simulink model "P1_LC"  (R2023b)
settings: Solver=VariableStepAuto  StartTime=0.0  StopTime=10.0  RelTol=1e-3
undefined symbols (not defined in the file): DiscIntNeverNeededParam
settings Model: Creator=Usuario_UMA  LastModifiedBy=pcele

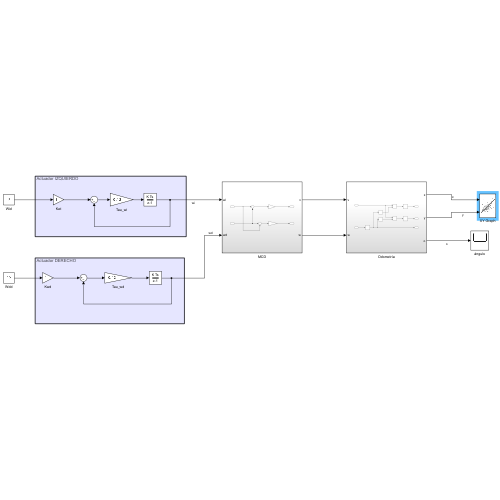
[thumbnail: Simulink's stored preview of the top-level diagram]
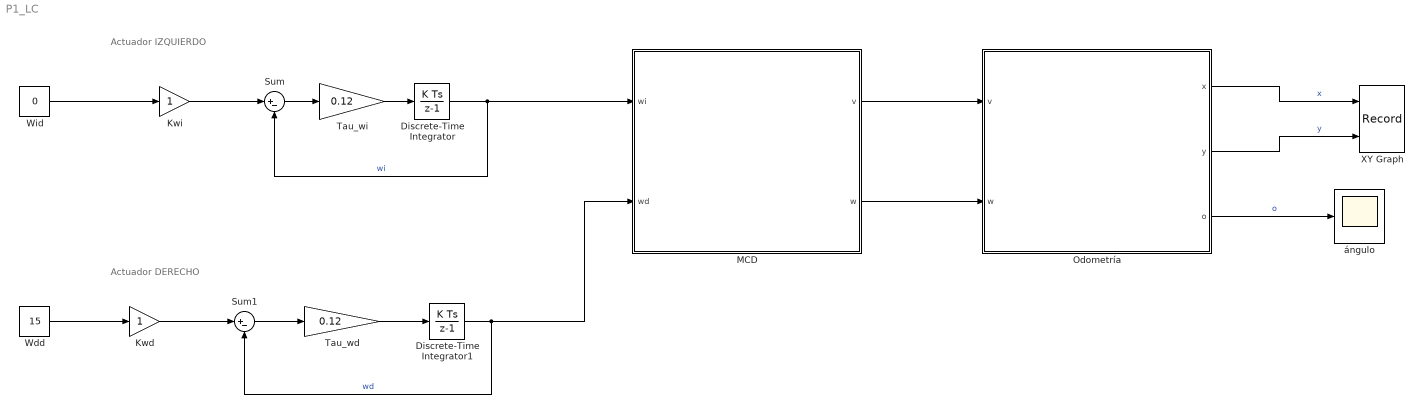
== system P1_LC ==
  note: Actuador IZQUIERDO
  note: Actuador DERECHO
  Discrete-Time Integrator : DiscreteIntegrator  SampleTime=0.25  ICPrevOutput=DiscIntNeverNeededParam  ICPrevScaledInput=DiscIntNeverNeededParam
  Discrete-Time Integrator1 : DiscreteIntegrator  SampleTime=0.25  ICPrevOutput=DiscIntNeverNeededParam  ICPrevScaledInput=DiscIntNeverNeededParam
  Kwd : Gain
  Kwi : Gain
  MCD : Subsystem
  Odometría : Subsystem
  Sum : Sum  Inputs=|+-
  Sum1 : Sum  Inputs=|+-
  Tau_wd : Gain  Gain=0.12
  Tau_wi : Gain  Gain=0.12
  Wdd : Constant  Value=15
  Wid : Constant  Value=0
  XY Graph : Record  FileSettingsInternal="{\"entries\":[{\"content\":{\"excelSettings\":{\"content\":{},\"type\":\"Streamout.ExcelSettings\"}},\"type\":\"Streamout.FileSettingStorage\",\"uuid\":\"\"}],\"packageUris\":[\"http:\\/\\/schema.mathworks.com\\/mf0\\/streamout_blocks\\/R2020a\"],\"version\":\"1.0\"}"  Layout=[1 1]  SignalsInternal="{\"entries\":[{\"content\":{\"signals\":[{\"content\":{\"blockPath\":[],\"dimensions\":[1],\"domain\":\"\",\"lineColor\":\"#a2142f\",\"plots\":[ 1 ],\"port\":1,\"sid\":[\"\"],\"signalID\":1,\"signalName\":\"x\"},\"type\":\"RecordBlkView.Signal\",\"uuid\":\"\"},{\"content\":{\"blockPath\":[],\"dimensions\":[1],\"domain\":\"\",\"lineColor\":\"#139fff\",\"plots\":[ 1 ],\"port\":2,\"sid\":[\"\"],\"signalID\":2,\"signalName\":\"y\"},\"type\":\"RecordBlkView.Signal\",\"uuid\":\"\"}]},\"type\":\"RecordBlkView.InputSignals\",\"uuid\":\"\"}],\"packageUris\":[\"http:\\/\\/schema.mathworks.com\\/mf0\\/streamout_blocks\\/R2020a\"],\"version\":\"1.0\"}"  VisualizationBindings="{\"xyplotplugin\":{\"info\":[{\"series\":[{\"bindingParametersList\":[{\"parameter\":\"X-Axis\",\"signalID\":1,\"signalName\":\"x\"},{\"parameter\":\"Y-Axis\",\"signalID\":2,\"signalName\":\"y\"}],\"seriesID\":0}],\"subplotID\":1}]}}"  CompatibilityTag=XY
  ángulo : Scope
  wires:
  Wid/1 -> Kwi/1
  Kwi/1 -> Sum/1
  Wdd/1 -> Kwd/1
  Kwd/1 -> Sum1/1
  Discrete-Time Integrator1/1 -> MCD/2(wd), Sum1/2  "wd"
  Sum1/1 -> Tau_wd/1
  Sum/1 -> Tau_wi/1
  Tau_wi/1 -> Discrete-Time Integrator/1
  Tau_wd/1 -> Discrete-Time Integrator1/1
  Discrete-Time Integrator/1 -> MCD/1(wi), Sum/2  "wi"
  MCD/1(v) -> Odometría/1(v)
  MCD/2(w) -> Odometría/2(w)
  Odometría/3(o) -> ángulo/1  "o"
  Odometría/1(x) -> XY Graph/1  "x"
  Odometría/2(y) -> XY Graph/2  "y"

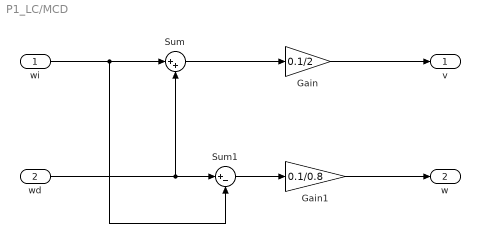
== system P1_LC/MCD ==
  wi : Inport
  wd : Inport  Port=2
  Gain : Gain  Gain=0.1/2
  Gain1 : Gain  Gain=0.1/0.8
  Sum : Sum  Inputs=|++
  Sum1 : Sum  Inputs=|+-
  v : Outport
  w : Outport  Port=2
  wires:
  Sum1/1 -> Gain1/1
  wd/1 -> Sum/2, Sum1/1
  wi/1 -> Sum1/2, Sum/1
  Sum/1 -> Gain/1
  Gain/1 -> v/1
  Gain1/1 -> w/1

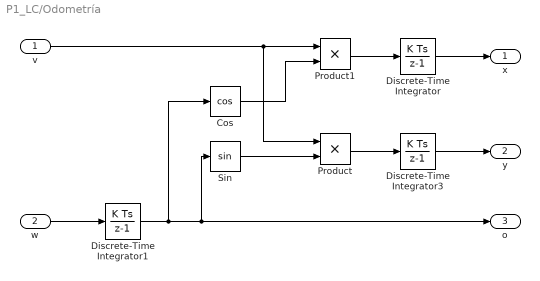
== system P1_LC/Odometría ==
  v : Inport
  w : Inport  Port=2
  Cos : Trigonometry  Operator=cos
  Discrete-Time Integrator : DiscreteIntegrator  SampleTime=0.25  ICPrevOutput=DiscIntNeverNeededParam  ICPrevScaledInput=DiscIntNeverNeededParam
  Discrete-Time Integrator1 : DiscreteIntegrator  SampleTime=0.25  ICPrevOutput=DiscIntNeverNeededParam  ICPrevScaledInput=DiscIntNeverNeededParam
  Discrete-Time Integrator3 : DiscreteIntegrator  SampleTime=0.25  ICPrevOutput=DiscIntNeverNeededParam  ICPrevScaledInput=DiscIntNeverNeededParam
  Product : Product
  Product1 : Product
  Sin : Trigonometry
  x : Outport
  y : Outport  Port=2
  o : Outport  Port=3
  wires:
  Cos/1 -> Product1/2
  Product1/1 -> Discrete-Time Integrator/1
  Discrete-Time Integrator/1 -> x/1
  v/1 -> Product/1, Product1/1
  w/1 -> Discrete-Time Integrator1/1
  Discrete-Time Integrator1/1 -> Sin/1, o/1, Cos/1
  Sin/1 -> Product/2
  Discrete-Time Integrator3/1 -> y/1
  Product/1 -> Discrete-Time Integrator3/1
